simulink model "projectFSR"  (R2023b)
settings: Solver=VariableStepAuto  StartTime=0.0  StopTime=150  RelTol=1e-3
libraries: robotmobilelib x2
settings Model: LastModifiedBy=vitto
settings ModelReferenceCC: EnableRefExpFcnMdlSchedulingChecks=on

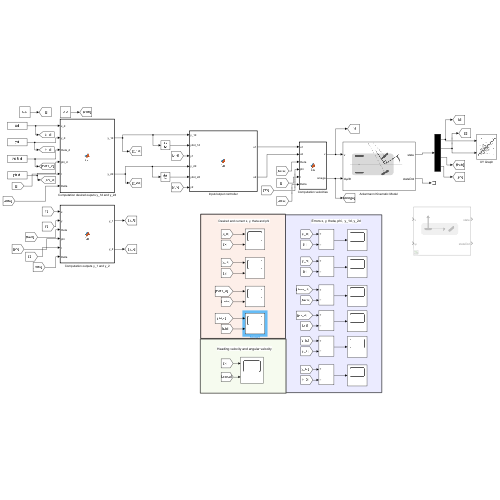
[thumbnail: Simulink's stored preview of the top-level diagram]
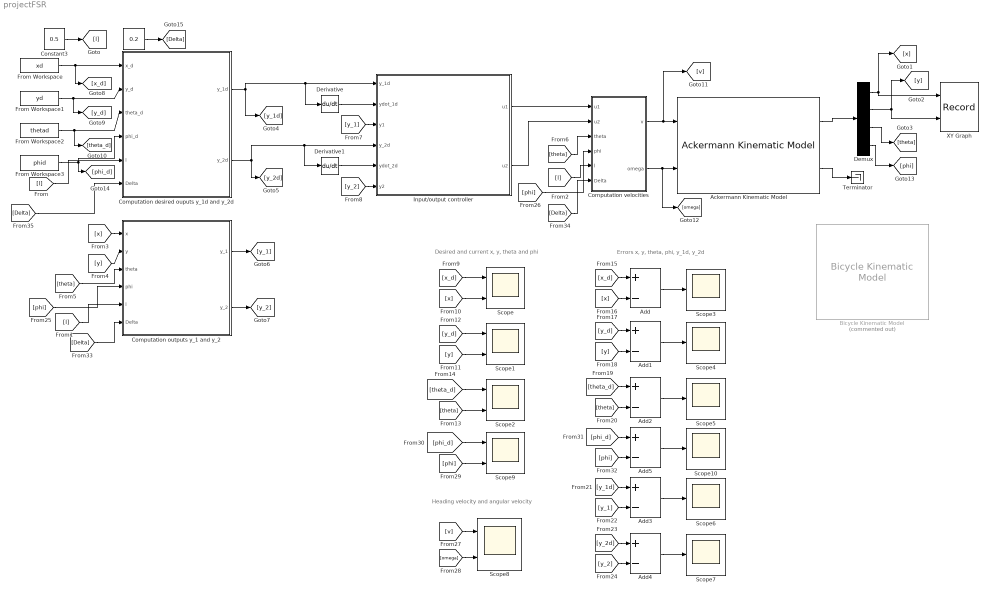
== system projectFSR ==
  note: Errors x, y, theta, phi, y_1d, y_2d
  note: Desired and current x, y, theta and phi
  note: Heading velocity and angular velocity
  " " : Constant  Value=0.2
  "Ackermann Kinematic Model " : robotmobilelib/Ackermann Kinematic Model  WheelBase=0.5  VehicleSpeedRange=[-inf inf]  MaxSteeringAngle=pi/4  InitialState=[30; 80; 0; 0]  SimulateUsing=Interpreted execution
  Add{,1..5} (6 alike) : Sum  Inputs=+-
  Bicycle Kinematic Model : robotmobilelib/Bicycle Kinematic Model  Commented=on  VehicleInputs=Vehicle Speed & Steering Angle  WheelBase=0.5  VehicleSpeedRange=[-inf inf]  MaxSteeringAngle=pi/4  InitialState=[0; 0; 0]  SimulateUsing=Interpreted execution
  Computation desired ouputs y_1d and y_2d : MATLAB Function  TreatAsAtomicUnit=on
  Computation outputs y_1 and y_2 : MATLAB Function  TreatAsAtomicUnit=on
  Computation velocities : MATLAB Function  TreatAsAtomicUnit=on
  Constant3 : Constant  Value=0.5
  Demux : Demux
  Derivative : Derivative
  Derivative1 : Derivative
  From Workspace : FromWorkspace  VariableName=xd
  From Workspace1 : FromWorkspace  VariableName=yd
  From Workspace2 : FromWorkspace  VariableName=thetad
  From Workspace3 : FromWorkspace  VariableName=phid
  Input/output controller : MATLAB Function  TreatAsAtomicUnit=on
  Scope{,1..2,8..9} (5 alike) : Scope  NumInputPorts=2
  Scope{3..7,10} (6 alike) : Scope
  Terminator : Terminator
  XY Graph : Record  FileSettingsInternal="{\"entries\":[{\"content\":{\"excelSettings\":{\"content\":{},\"type\":\"Streamout.ExcelSettings\"}},\"type\":\"Streamout.FileSettingStorage\",\"uuid\":\"\"}],\"packageUris\":[\"http:\\/\\/schema.mathworks.com\\/mf0\\/streamout_blocks\\/R2020a\"],\"version\":\"1.0\"}"  Layout=[1 1]  SignalsInternal="{\"entries\":[{\"content\":{\"signals\":[{\"content\":{\"blockPath\":[],\"dimensions\":[1],\"domain\":\"\",\"lineColor\":\"#a2142f\",\"plots\":[1],\"port\":1,\"sid\":[\"\"],\"signalID\":1007,\"signalName\":\"Demux:1\"},\"type\":\"RecordBlkView.Signal\",\"uuid\":\"\"},{\"content\":{\"blockPath\":[],\"dimensions\":[1],\"domain\":\"\",\"lineColor\":\"#139fff\",\"plots\":[1],\"port\":2,\"sid\":[\"\"],\"signalID\":1011,\"signalName\":\"Demux:2\"},\"type\":\"RecordBlkView.Signal\",\"uuid\":\"\"}]},\"type\":\"RecordBlkView.InputSignals\",\"uuid\":\"\"}],\"packageUris\":[\"http:\\/\\/schema.mathworks.com\\/mf0\\/streamout_blocks\\/R2020a\"],\"version\":\"1.0\"}"  VisualizationBindings="{\"xyplotplugin\":{\"info\":[{\"series\":[{\"bindingParametersList\":[{\"parameter\":\"X-Axis\",\"signalID\":1007,\"signalName\":\"Demux:1\"},{\"parameter\":\"Y-Axis\",\"signalID\":1011,\"signalName\":\"Demux:2\"}],\"seriesID\":2048}],\"subplotID\":1}]}}"  CompatibilityTag=XY
  wires:
  Computation velocities/2(omega) -> "Ackermann Kinematic Model "/2, [omega]
  From Workspace/1 -> [x_d], Computation desired ouputs y_1d and y_2d/1(x_d)
  From Workspace1/1 -> [y_d], Computation desired ouputs y_1d and y_2d/2(y_d)
  From Workspace2/1 -> [theta_d], Computation desired ouputs y_1d and y_2d/3(theta_d)
  Constant3/1 -> [l]
  [l] -> Computation desired ouputs y_1d and y_2d/5(l)
  Computation desired ouputs y_1d and y_2d/1(y_1d) -> Derivative/1, Input/output controller/1(y_1d), [y_1d]
  Input/output controller/1(u1) -> Computation velocities/1(u1)
  Input/output controller/2(u2) -> Computation velocities/2(u2)
  [l] -> Computation outputs y_1 and y_2/5(l)
  [l] -> Computation velocities/5(l)
  Demux/3 -> [theta]
  [x] -> Computation outputs y_1 and y_2/1(x)
  [y] -> Computation outputs y_1 and y_2/2(y)
  [theta] -> Computation outputs y_1 and y_2/3(theta)
  [theta] -> Computation velocities/3(theta)
  Computation desired ouputs y_1d and y_2d/2(y_2d) -> Derivative1/1, Input/output controller/4(y_2d), [y_2d]
  Computation outputs y_1 and y_2/1(y_1) -> [y_1]
  Computation outputs y_1 and y_2/2(y_2) -> [y_2]
  [y_1] -> Input/output controller/3(y1)
  [y_2] -> Input/output controller/6(y2)
  [x_d] -> Scope/1
  [x] -> Scope/2
  [y_d] -> Scope1/1
  [y] -> Scope1/2
  [theta_d] -> Scope2/1
  [theta] -> Scope2/2
  [x_d] -> Add/1
  [x] -> Add/2
  Add/1 -> Scope3/1
  [y_d] -> Add1/1
  [y] -> Add1/2
  Add1/1 -> Scope4/1
  [theta_d] -> Add2/1
  [theta] -> Add2/2
  Add2/1 -> Scope5/1
  Add3/1 -> Scope6/1
  [y_1] -> Add3/2
  [y_1d] -> Add3/1
  Add4/1 -> Scope7/1
  [y_2] -> Add4/2
  [y_2d] -> Add4/1
  Demux/1 -> XY Graph/1, [x]
  Demux/2 -> XY Graph/2, [y]
  Computation velocities/1(v) -> [v], "Ackermann Kinematic Model "/1
  [v] -> Scope8/1
  [omega] -> Scope8/2
  Demux/4 -> [phi]
  [phi] -> Computation outputs y_1 and y_2/4(phi)
  From Workspace3/1 -> [phi_d], Computation desired ouputs y_1d and y_2d/4(phi_d)
  [phi] -> Computation velocities/4(phi)
  "Ackermann Kinematic Model "/1 -> Demux/1
  "Ackermann Kinematic Model "/2 -> Terminator/1
  [phi_d] -> Scope9/1
  [phi] -> Scope9/2
  Add5/1 -> Scope10/1
  [phi_d] -> Add5/1
  [phi] -> Add5/2
  Derivative1/1 -> Input/output controller/5(ydot_2d)
  Derivative/1 -> Input/output controller/2(ydot_1d)
  " "/1 -> [Delta]
  [Delta] -> Computation outputs y_1 and y_2/6(Delta)
  [Delta] -> Computation velocities/6(Delta)
  [Delta] -> Computation desired ouputs y_1d and y_2d/6(Delta)

== matlab function projectFSR/Computation desired ouputs y_1d and y_2d ==
  data: x_d input; y_1d output; y_d input; theta_d input; phi_d input; y_2d output; l input; Delta input
function [y_1d, y_2d]  = fcn(x_d, y_d, theta_d, phi_d, l, Delta)

y_1d = x_d+l*cos(theta_d)+Delta*cos(theta_d+phi_d);
y_2d = y_d+l*sin(theta_d)+Delta*sin(theta_d+phi_d);
 
end

== matlab function projectFSR/Computation velocities ==
  data: u1 input; v output; omega output; u2 input; theta input; phi input; l input; Delta input
function [v, omega] = fcn(u1, u2, theta, phi, l, Delta)

A = [cos(theta)-tan(phi)*(sin(theta)+(Delta*sin(theta+phi))/l) -Delta*sin(theta+phi);
     sin(theta)+tan(phi)*(cos(theta)+(Delta*cos(theta+phi))/l) +Delta*cos(theta+phi)];

Ainv = inv(A);

v = Ainv(1,:)*[u1; u2];
omega = Ainv(2,:)*[u1; u2];


end

== matlab function projectFSR/Input//output controller ==
  data: y_1d input; u1 output; ydot_1d input; y1 input; y_2d input; ydot_2d input; y2 input; u2 output
function [u1, u2] = fcn(y_1d, ydot_1d, y1, y_2d, ydot_2d, y2)

k1 = 2; %6  %10
k2 = 2; %6  %10

u1 = ydot_1d+k1*(y_1d-y1);
u2 = ydot_2d+k2*(y_2d-y2);

end

== matlab function projectFSR/Computation outputs y_1 and y_2 ==
  data: x input; y_1 output; y input; theta input; phi input; y_2 output; l input; Delta input
function [y_1, y_2]  = fcn(x, y, theta, phi, l, Delta)

y_1 = x+l*cos(theta)+Delta*cos(theta+phi);
y_2 = y+l*sin(theta)+Delta*sin(theta+phi);

end
